simulink model "Remedy_WWTP_OL_FMU_2021b"  (R2021b)
settings: Solver=ode23tb  StartTime=0.0  StopTime=100  FixedStep=1E-4  MaxStep=100  RelTol=1e-3  EnableMultiTasking=on
settings Model: SimulationMode=rapid-accelerator  Creator=iirizar  LastModifiedBy=ion
settings SolverCC: InitialStep=1E-22  MaxConsecutiveMinStep=auto  AlgebraicLoopSolver=TrustRegion
settings DataIOCC: MaxDataPoints=1  SaveFormat=Array  SignalLoggingSaveFormat=ModelDataLogs  SaveOutput=off  SignalLogging=off  DSMLogging=off  SaveTime=off  ReturnWorkspaceOutputs=off
settings OptimizationCC: DefaultParameterBehavior=Inlined  GainParamInheritBuiltInType=on  UseFloatMulNetSlope=on  InlineInvariantSignals=on  ExpressionDepthLimit=2147483647  EfficientFloat2IntCast=on
settings DebuggingCC: UnderspecifiedInitializationDetection=Classic  MergeDetectMultiDrivingBlocksExec=none  SolverPrmCheckMsg=warning  FcnCallInpInsideContextMsg=warning  UnconnectedOutputMsg=none  UnconnectedLineMsg=none  StateNameClashWarn=warning  SFUnexpectedBacktrackingDiag=warning  SFNoUnconditionalDefaultTransitionDiag=warning  SFExecutionAtInitializationDiag=none  SFMachineParentedDataDiag=warning  ArithmeticOperatorsInVariantConditions=warning
settings HardwareCC: TargetBitPerPointer=64  TargetBitPerSizeT=64  TargetBitPerPtrDiffT=64  TargetLongLongMode=on  TargetIntDivRoundTo=Zero  TargetEndianess=LittleEndian  TargetWordSize=64  TargetHWDeviceType=MATLAB Host  ProdEqTarget=off
settings ModelReferenceCC: ModelReferenceMinAlgLoopOccurrences=on  PropagateSignalLabelsOutOfModel=off
settings SFSimCC: SimUseLocalCustomCode=off  CustomCodeUndefinedFunction=UseInterfaceOnly
settings RTWCC: Description=FMU based on RTW S-Function (Functional Mock-up Unit)  SystemTargetFile=rtwsfcnfmi.tlc  GenerateMakefile=off  TemplateMakefile=none  RetainRTWFile=on  RTWUseLocalCustomCode=off  BuildConfiguration=Faster Runs  DLArmComputeVersion=20.02.1
settings CodeAppCC: ForceParamTrailComments=on  StateflowObjectComments=on
settings STFCustomTargetCC: ModelReferenceCompliant=off  CompOptLevelCompliant=on  MATLABClassNameForMDSCustomization=Simulink.SoftwareTarget.TargetSpecificTriggerConfigurationBase  SystemTargetFile=rtwsfcnfmi.tlc
settings ConfigComp: CovMetricSettings=dw  CovSaveCumulativeToWorkspaceVar=on  CovSaveSingleToWorkspaceVar=on  CovExternalEMLEnable=off

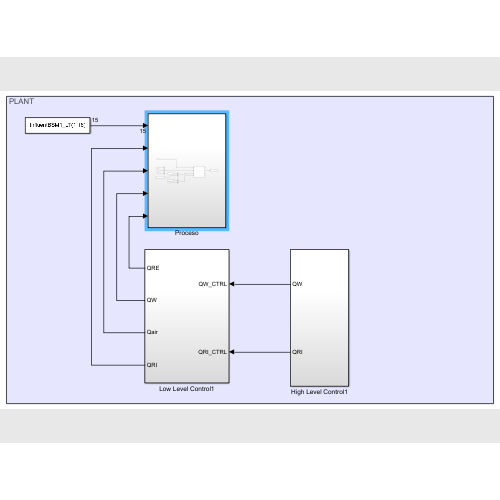
[thumbnail: Simulink's stored preview of the top-level diagram]
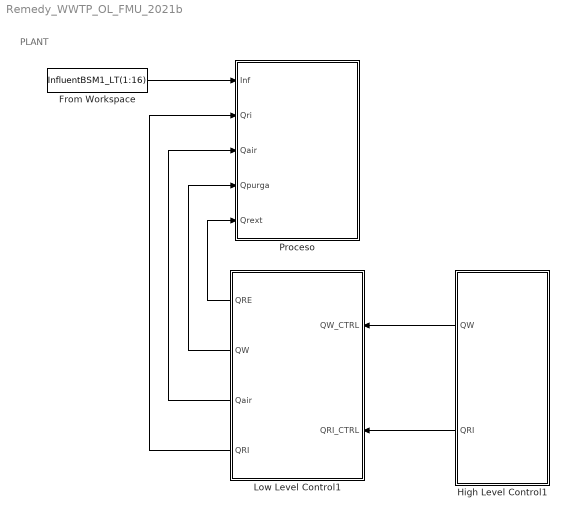
== system Remedy_WWTP_OL_FMU_2021b ==
  note: PLANT
  From Workspace : FromWorkspace  VariableName=InfluentBSM1_LT(1:16)  OutputAfterFinalValue=Holding final value
  High Level Control1 : Subsystem
  Low Level Control1 : Subsystem
  Proceso : Subsystem
  wires:
  Low Level Control1/2(QW) -> Proceso/4(Qpurga)
  Low Level Control1/3(Qair) -> Proceso/3(Qair)
  Low Level Control1/1(QRE) -> Proceso/5(Qrext)
  High Level Control1/2(QRI) -> Low Level Control1/2(QRI_CTRL)
  High Level Control1/1(QW) -> Low Level Control1/1(QW_CTRL)
  Low Level Control1/4(QRI) -> Proceso/2(Qri)
  From Workspace/1 -> Proceso/1(Inf)

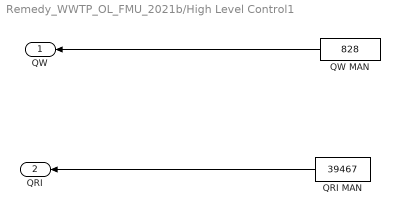
== system Remedy_WWTP_OL_FMU_2021b/High Level Control1 ==
  QRI MAN : Constant  Value=39467
  QW MAN : Constant  Value=828
  QW : Outport
  QRI : Outport  Port=2
  wires:
  QRI MAN/1 -> QRI/1
  QW MAN/1 -> QW/1

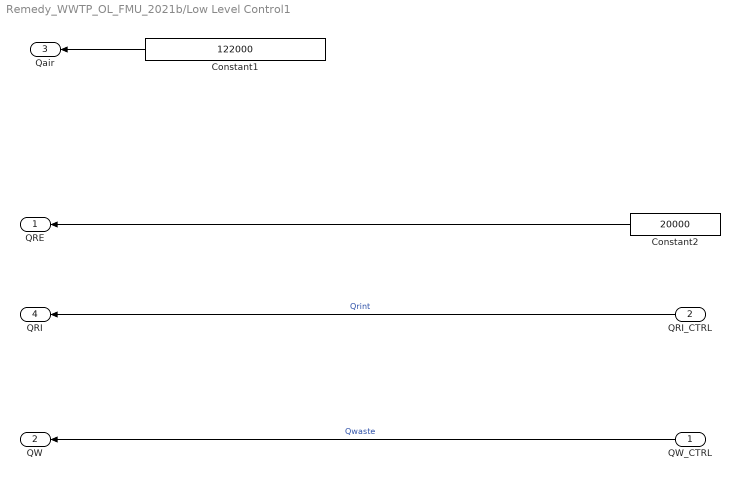
== system Remedy_WWTP_OL_FMU_2021b/Low Level Control1 ==
  QW_CTRL : Inport
  QRI_CTRL : Inport  Port=2
  Constant1 : Constant  Value=122000
  Constant2 : Constant  Value=20000
  QRE : Outport
  QW : Outport  Port=2
  Qair : Outport  Port=3
  QRI : Outport  Port=4
  wires:
  QRI_CTRL/1 -> QRI/1  "Qrint"
  QW_CTRL/1 -> QW/1  "Qwaste"
  Constant2/1 -> QRE/1
  Constant1/1 -> Qair/1

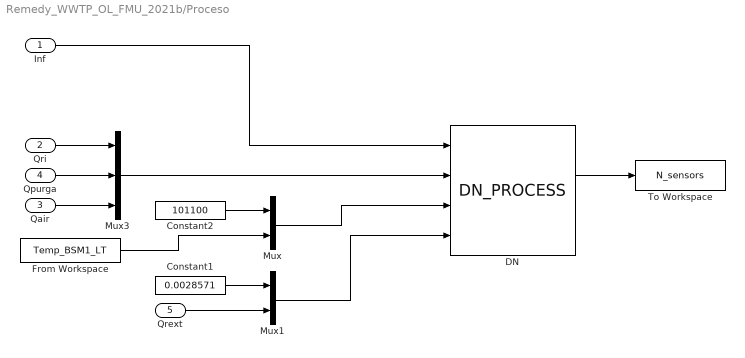
== system Remedy_WWTP_OL_FMU_2021b/Proceso ==
  Inf : Inport
  Qri : Inport  Port=2
  Qair : Inport  Port=3
  Qpurga : Inport  Port=4
  Qrext : Inport  Port=5
  Constant1 : Constant  Value=0.0028571
  Constant2 : Constant  Value=101100
  DN : S-Function  FunctionName=DN_PROCESS  Parameters=ParamsEsteq,Cineticos20,Arrhenius,Esteq, Param_D,Param_N, x0  SFunctionDeploymentMode=off  EnableBusSupport=off
      mask Display: image('$imagefile'); % Use "Edit Image" on toolstrip to change.
  From Workspace : FromWorkspace  VariableName=Temp_BSM1_LT  OutputAfterFinalValue=Holding final value
  Mux : Mux  Inputs=2
  Mux1 : Mux  Inputs=2
  Mux3 : Mux  Inputs=3
  To Workspace : ToWorkspace  VariableName=N_sensors  SampleTime=15/1440
      settings: MaxDataPoints=100
  wires:
  Qri/1 -> Mux3/1
  Inf/1 -> DN/1
  Qpurga/1 -> Mux3/2
  Qair/1 -> Mux3/3
  Mux3/1 -> DN/2
  Mux/1 -> DN/3
  Qrext/1 -> Mux1/2
  Mux1/1 -> DN/4
  Constant2/1 -> Mux/1
  Constant1/1 -> Mux1/1
  From Workspace/1 -> Mux/2
  DN/2 -> To Workspace/1
